simulink model "TSR_Scenario_002_cs"  (R2014b)
settings: Solver=ode5  SolverMode=SingleTasking  StartTime=0.0  StopTime=inf  FixedStep=1/100  RelTol=1e-3
PreLoadFcn:
  | mbxruntime.callbacks.PreLoadFcn(bdroot);
  | check_NUTS_defined;
  | 
  | assignin('base',['model_closed_' bdroot],false);
  | 
  | addpath('../includes_TSR/includes_TSR');
  | 
  | switch version('-release')
  | case {'2010a', '2010b', '2011a'}
  | addpath('../includes_TSR/ML2010b');
  | otherwise
  | addpath('../includes_TSR/ML2011b');
  | end
PostLoadFcn:
  | mbxruntime.callbacks.PostLoadFcn(bdroot);
InitFcn:
  | mbxruntime.callbacks.InitFcn(bdroot);;
  | 
  | addpath('..\includes_TSR');
StartFcn:
  | mbxruntime.callbacks.StartFcn(bdroot);
StopFcn:
  | mbxruntime.callbacks.StopFcn(bdroot);
model workspace: external: MAT-File .\TSR_Scenario_002_cs_hws.mat (data not in the file)
undefined symbols (not defined in the file or in its folder): InitImageOutputDir, mbxruntime, OrientationPitch, OrientationRoll, PositionX, PositionY, PositionZ, tabledata, warningInitialVelocity, x0
undefined symbols (not defined in the file): SteeringColumn, SteeringWheel, TSR_Scenario_002_cs_003e47b1b59594b6, TSR_Scenario_002_cs_023e87a31011dc74, TSR_Scenario_002_cs_048cb8409c90d9c6, TSR_Scenario_002_cs_106a0284aafa53e6, TSR_Scenario_002_cs_195b368d22a7f172, TSR_Scenario_002_cs_1e339fa5d680f213, TSR_Scenario_002_cs_26196a9fb104f950, TSR_Scenario_002_cs_261a709f6f453598, TSR_Scenario_002_cs_2ac3337370d0049d, TSR_Scenario_002_cs_2dc51e6a68b01b00, TSR_Scenario_002_cs_3460ff54d38ab2e2, TSR_Scenario_002_cs_42ea7d6e56bd6005, TSR_Scenario_002_cs_4dd419d6d2b56fc2, TSR_Scenario_002_cs_5316a21de09dff2f, TSR_Scenario_002_cs_538caacf3455966d, TSR_Scenario_002_cs_5b2cfdbcfc80811f, TSR_Scenario_002_cs_5ce0eafbb7a2dce7, TSR_Scenario_002_cs_62cdbf45c6f8824a, TSR_Scenario_002_cs_6bebc368eedff0bc, TSR_Scenario_002_cs_6d26481da4ed7e29, TSR_Scenario_002_cs_70c7e369ce6550e0, TSR_Scenario_002_cs_7a63051a1f311451, TSR_Scenario_002_cs_7d7dc8405f613c6d, TSR_Scenario_002_cs_7f65e296173485e8, TSR_Scenario_002_cs_87183cf6ff7bb4b6, TSR_Scenario_002_cs_8921b0da7ab80865, TSR_Scenario_002_cs_9495ce3a76763d1f, TSR_Scenario_002_cs_a679806a2fdc8099, TSR_Scenario_002_cs_Actros_1860_1_Path_pathUniqueID, TSR_Scenario_002_cs_Actros_2541_1_Path_pathUniqueID, TSR_Scenario_002_cs_Actros_2541_3_Path_pathUniqueID, TSR_Scenario_002_cs_Actros_2541_4_Path_pathUniqueID, TSR_Scenario_002_cs_adf24c93a9de8a4e, TSR_Scenario_002_cs_Audi_A8_1_Dynamics_Simple_initialPitch, TSR_Scenario_002_cs_Audi_A8_1_Dynamics_Simple_initialRoll, TSR_Scenario_002_cs_Audi_A8_1_Dynamics_Simple_initialX, TSR_Scenario_002_cs_Audi_A8_1_Dynamics_Simple_initialY, TSR_Scenario_002_cs_Audi_A8_1_Dynamics_Simple_initialYaw, TSR_Scenario_002_cs_Audi_A8_1_Dynamics_Simple_initialZ, TSR_Scenario_002_cs_b136c6ccb55f77db, TSR_Scenario_002_cs_ba4f809714c282b7, TSR_Scenario_002_cs_BMW_X5_1_Path_pathUniqueID, TSR_Scenario_002_cs_BMW_X5_1_SpeedProfile_speedProfileUniqueID, TSR_Scenario_002_cs_BMW_X5_2_Path_pathUniqueID, TSR_Scenario_002_cs_BMW_X5_2_SpeedProfile_speedProfileUniqueID, TSR_Scenario_002_cs_Citroen_C3_1_Path_pathUniqueID, TSR_Scenario_002_cs_Citroen_C3_2_Path_pathUniqueID, TSR_Scenario_002_cs_d8f275339b7082cf, TSR_Scenario_002_cs_Daf_95_1_Path_pathUniqueID, TSR_Scenario_002_cs_Daf_95_1_SpeedProfile_speedProfileUniqueID, TSR_Scenario_002_cs_dc019741510ce2f2, TSR_Scenario_002_cs_fdbc8aabe460b27c, TSR_Scenario_002_cs_Fiat_Bravo_1_Path_pathUniqueID, TSR_Scenario_002_cs_Ford_Fiesta_1_Path_pathUniqueID, TSR_Scenario_002_cs_Honda_Pan_European_1_Path_pathUniqueID, TSR_Scenario_002_cs_Mazda_RX8_1_Path_pathUniqueID, TSR_Scenario_002_cs_Nissan_Cabstar_1_Path_pathUniqueID, TSR_Scenario_002_cs_Nissan_Cabstar_2_Path_pathUniqueID ... (+9)
libraries: simulink_extras x82, simulink x23, PreScanSimulinkLibrary x11
(part 21 of 39)

== system TSR_Scenario_002_cs/HighwayOverhang_6/VISUMatrixSign_Mux ==
  MatrixSign_19 : Inport
  MatrixSign_20 : Inport  Port=2
  MatrixSign_19_Conversion : DataTypeConversion
  MatrixSign_19_InitialResource : Constant
  MatrixSign_19_Switch : Switch  Criteria=u2 ~= 0
  MatrixSign_20_Conversion : DataTypeConversion
  MatrixSign_20_InitialResource : Constant
  MatrixSign_20_Switch : Switch  Criteria=u2 ~= 0
  SubMuxMatrixSign : Mux  Inputs=2
  MatrixSigns : Outport
  wires:
  SubMuxMatrixSign/1 -> MatrixSigns/1
  MatrixSign_19/1 -> MatrixSign_19_Switch/1, MatrixSign_19_Switch/2
  MatrixSign_19_InitialResource/1 -> MatrixSign_19_Switch/3
  MatrixSign_19_Switch/1 -> MatrixSign_19_Conversion/1
  MatrixSign_19_Conversion/1 -> SubMuxMatrixSign/1
  MatrixSign_20/1 -> MatrixSign_20_Switch/1, MatrixSign_20_Switch/2
  MatrixSign_20_InitialResource/1 -> MatrixSign_20_Switch/3
  MatrixSign_20_Switch/1 -> MatrixSign_20_Conversion/1
  MatrixSign_20_Conversion/1 -> SubMuxMatrixSign/2

== system TSR_Scenario_002_cs/HighwayOverhang_7/VISUMatrixSignLights_Mux ==
  MatrixSign_4 : Inport  Tag=inport/MatrixSign_4  PortDimensions=4  SampleTime=1/100  BusOutputAsStruct=on
  MatrixSign_45 : Inport  Tag=inport/MatrixSign_45  Port=2  PortDimensions=4  SampleTime=1/100  BusOutputAsStruct=on
  MuxVisuLights : Mux  Inputs=2
  VISUMatrixSignLights_HighwayOverhang_7 : Outport  Tag=outport/VisuMatrixSignLights  SampleTime=1/100
  wires:
  MuxVisuLights/1 -> VISUMatrixSignLights_HighwayOverhang_7/1
  MatrixSign_4/1 -> MuxVisuLights/1
  MatrixSign_45/1 -> MuxVisuLights/2

== system TSR_Scenario_002_cs/HighwayOverhang_7/VISUMatrixSign_Mux ==
  MatrixSign_4 : Inport
  MatrixSign_45 : Inport  Port=2
  MatrixSign_45_Conversion : DataTypeConversion
  MatrixSign_45_InitialResource : Constant  Value=15
  MatrixSign_45_Switch : Switch  Criteria=u2 ~= 0
  MatrixSign_4_Conversion : DataTypeConversion
  MatrixSign_4_InitialResource : Constant  Value=15
  MatrixSign_4_Switch : Switch  Criteria=u2 ~= 0
  SubMuxMatrixSign : Mux  Inputs=2
  MatrixSigns : Outport
  wires:
  SubMuxMatrixSign/1 -> MatrixSigns/1
  MatrixSign_4/1 -> MatrixSign_4_Switch/1, MatrixSign_4_Switch/2
  MatrixSign_4_InitialResource/1 -> MatrixSign_4_Switch/3
  MatrixSign_4_Switch/1 -> MatrixSign_4_Conversion/1
  MatrixSign_4_Conversion/1 -> SubMuxMatrixSign/1
  MatrixSign_45/1 -> MatrixSign_45_Switch/1, MatrixSign_45_Switch/2
  MatrixSign_45_InitialResource/1 -> MatrixSign_45_Switch/3
  MatrixSign_45_Switch/1 -> MatrixSign_45_Conversion/1
  MatrixSign_45_Conversion/1 -> SubMuxMatrixSign/2

== system TSR_Scenario_002_cs/HighwayOverhang_8/VISUMatrixSignLights_Mux ==
  MatrixSign_15 : Inport  Tag=inport/MatrixSign_15  PortDimensions=4  SampleTime=1/100  BusOutputAsStruct=on
  MatrixSign_16 : Inport  Tag=inport/MatrixSign_16  Port=2  PortDimensions=4  SampleTime=1/100  BusOutputAsStruct=on
  MuxVisuLights : Mux  Inputs=2
  VISUMatrixSignLights_HighwayOverhang_8 : Outport  Tag=outport/VisuMatrixSignLights  SampleTime=1/100
  wires:
  MuxVisuLights/1 -> VISUMatrixSignLights_HighwayOverhang_8/1
  MatrixSign_15/1 -> MuxVisuLights/1
  MatrixSign_16/1 -> MuxVisuLights/2

== system TSR_Scenario_002_cs/HighwayOverhang_8/VISUMatrixSign_Mux ==
  MatrixSign_15 : Inport
  MatrixSign_16 : Inport  Port=2
  MatrixSign_15_Conversion : DataTypeConversion
  MatrixSign_15_InitialResource : Constant
  MatrixSign_15_Switch : Switch  Criteria=u2 ~= 0
  MatrixSign_16_Conversion : DataTypeConversion
  MatrixSign_16_InitialResource : Constant
  MatrixSign_16_Switch : Switch  Criteria=u2 ~= 0
  SubMuxMatrixSign : Mux  Inputs=2
  MatrixSigns : Outport
  wires:
  SubMuxMatrixSign/1 -> MatrixSigns/1
  MatrixSign_15/1 -> MatrixSign_15_Switch/1, MatrixSign_15_Switch/2
  MatrixSign_15_InitialResource/1 -> MatrixSign_15_Switch/3
  MatrixSign_15_Switch/1 -> MatrixSign_15_Conversion/1
  MatrixSign_15_Conversion/1 -> SubMuxMatrixSign/1
  MatrixSign_16/1 -> MatrixSign_16_Switch/1, MatrixSign_16_Switch/2
  MatrixSign_16_InitialResource/1 -> MatrixSign_16_Switch/3
  MatrixSign_16_Switch/1 -> MatrixSign_16_Conversion/1
  MatrixSign_16_Conversion/1 -> SubMuxMatrixSign/2

== system TSR_Scenario_002_cs/HighwayOverhang_9/VISUMatrixSignLights_Mux ==
  MatrixSign_47 : Inport  Tag=inport/MatrixSign_47  PortDimensions=4  SampleTime=1/100  BusOutputAsStruct=on
  MatrixSign_6 : Inport  Tag=inport/MatrixSign_6  Port=2  PortDimensions=4  SampleTime=1/100  BusOutputAsStruct=on
  MuxVisuLights : Mux  Inputs=2
  VISUMatrixSignLights_HighwayOverhang_9 : Outport  Tag=outport/VisuMatrixSignLights  SampleTime=1/100
  wires:
  MuxVisuLights/1 -> VISUMatrixSignLights_HighwayOverhang_9/1
  MatrixSign_47/1 -> MuxVisuLights/1
  MatrixSign_6/1 -> MuxVisuLights/2

== system TSR_Scenario_002_cs/HighwayOverhang_9/VISUMatrixSign_Mux ==
  MatrixSign_6 : Inport
  MatrixSign_47 : Inport  Port=2
  MatrixSign_47_Conversion : DataTypeConversion
  MatrixSign_47_InitialResource : Constant  Value=13
  MatrixSign_47_Switch : Switch  Criteria=u2 ~= 0
  MatrixSign_6_Conversion : DataTypeConversion
  MatrixSign_6_InitialResource : Constant  Value=13
  MatrixSign_6_Switch : Switch  Criteria=u2 ~= 0
  SubMuxMatrixSign : Mux  Inputs=2
  MatrixSigns : Outport
  wires:
  SubMuxMatrixSign/1 -> MatrixSigns/1
  MatrixSign_6/1 -> MatrixSign_6_Switch/1, MatrixSign_6_Switch/2
  MatrixSign_6_InitialResource/1 -> MatrixSign_6_Switch/3
  MatrixSign_6_Switch/1 -> MatrixSign_6_Conversion/1
  MatrixSign_6_Conversion/1 -> SubMuxMatrixSign/1
  MatrixSign_47/1 -> MatrixSign_47_Switch/1, MatrixSign_47_Switch/2
  MatrixSign_47_InitialResource/1 -> MatrixSign_47_Switch/3
  MatrixSign_47_Switch/1 -> MatrixSign_47_Conversion/1
  MatrixSign_47_Conversion/1 -> SubMuxMatrixSign/2

== system TSR_Scenario_002_cs/Honda_Pan_European_1/SELF_Demux ==
  SELF : Inport  OutDataTypeStr=Bus: PRESCAN_SELFSENSORDATA
  Bus Selector : BusSelector  OutputSignals=PositionX,PositionY,PositionZ,OrientationRoll,OrientationPitch,OrientationYaw,Velocity,Yaw_rate,Lat,Long,Alt
  Demux2 : Demux  Outputs=3
  Gain : Gain  Gain=180/pi
  Gain1 : Gain  Gain=180/pi
  Vector Concatenate1 : Concatenate  NumInputs=3
  compas converter : Subsystem
  x [m] : Outport
  y [m] : Outport  Port=2
  z [m] : Outport  Port=3
  rotx [deg] : Outport  Port=4
  roty [deg] : Outport  Port=5
  rotz [deg] : Outport  Port=6
  GPS lat [deg] : Outport  Port=7
  GPS long [deg] : Outport  Port=8
  GPS alt [m] : Outport  Port=9
  velocity [m/s] : Outport  Port=10
  heading [deg] : Outport  Port=11
  yaw rate [deg/s] : Outport  Port=12
  wires:
  Bus Selector/11 -> GPS alt [m]/1  "<Alt>"
  Bus Selector/10 -> GPS long [deg]/1  "<Long>"
  Bus Selector/9 -> GPS lat [deg]/1  "<Lat>"
  Bus Selector/8 -> Gain1/1  "<Yaw_rate>"
  Bus Selector/7 -> velocity [m/s]/1  "<Velocity>"
  Bus Selector/6 -> compas converter/1(rotz [rad]), Vector Concatenate1/3  "<OrientationYaw>"
  Bus Selector/5 -> Vector Concatenate1/2  "<OrientationPitch>"
  Bus Selector/4 -> Vector Concatenate1/1  "<OrientationRoll>"
  Vector Concatenate1/1 -> Gain/1
  Bus Selector/3 -> z [m]/1  "<PositionZ>"
  Bus Selector/2 -> y [m]/1  "<PositionY>"
  Bus Selector/1 -> x [m]/1  "<PositionX>"
  SELF/1 -> Bus Selector/1
  Gain/1 -> Demux2/1
  Demux2/1 -> rotx [deg]/1
  Demux2/2 -> roty [deg]/1
  Demux2/3 -> rotz [deg]/1
  compas converter/1(heading [deg]) -> heading [deg]/1
  Gain1/1 -> yaw rate [deg/s]/1

== system TSR_Scenario_002_cs/Male_RegularAni_1/Animation ==
  In1 : Inport
  Bus Creator : BusCreator  Inputs=2  OutDataTypeStr=Bus: PRESCAN_ANIMACTUATORDATA  NonVirtualBus=on
  Bus Selector : BusSelector  OutputSignals=VelocityX,VelocityY,VelocityZ
  Data Type Conversion : DataTypeConversion  OutDataTypeStr=int32
  Mux : Mux  Inputs=3
  Product : Product  RndMeth=Zero
  RunningScale : Constant  Value=RunningScale
  Switch : Switch  Threshold=2
  WalkingScale : Constant  Value=WalkingScale
  animation mode : Subsystem
  elapsed track : Subsystem
  Out1 : Outport
  wires:
  Switch/1 -> Product/1
  WalkingScale/1 -> Switch/3
  RunningScale/1 -> Switch/1
  elapsed track/1(s) -> Product/2  "Time"
  Product/1 -> Bus Creator/2  "Time"
  Mux/1 -> elapsed track/1(vel), animation mode/1(vel)
  Bus Selector/1 -> Mux/1  "<VelocityX>"
  Bus Selector/2 -> Mux/2  "<VelocityY>"
  Bus Selector/3 -> Mux/3  "<VelocityZ>"
  animation mode/1(mode) -> Switch/2, Data Type Conversion/1
  In1/1 -> Bus Selector/1
  Bus Creator/1 -> Out1/1
  Data Type Conversion/1 -> Bus Creator/1  "Index"

== system TSR_Scenario_002_cs/Male_RegularAni_1/Dynamics_Empty ==
  note: For state mode 'Dynamic' positions
      | are not taken into account, as they
      | are computed by integrating velocity.
      | Click annotation for Help.
  Ground_{1..9} (9 alike) : Ground
  MuxState : Subsystem  Tag=mux/State  mask(Empty Dynamics State Block){positioningmode=on, TimeStep=1/100}
      mask prompts: positioningmode "Positioning Mode"; TimeStep "Auto Assigned: Time Step [s]"
      mask help:
      | Build the state of an actor based on user input.
      | The user can either use positioning mode or dynamics mode.
      | - When using positioning mode the position and orientation of the actor are set directly based on the input. Expected input is relative to the initial position and orientation of the actor. It's also possible to specify the velocity of the actor, though this input isn't used, only passed on.
      | - When using dynamics mode the position input is ignored. Expected input is velocity and orientation. The velocity is relative the current orientation of the actor, while orientation is relative to its initial orientation. The position of the actor is calculated based on the velocity and orientation given.
      settings: DeleteFcn=PreScanBlockDeleteFcn;
  STATE_Male_RegularAni_1 : Subsystem  Tag=mux/StatePort  Priority=0  LoadFcn=load PrescanStateActuatorData  mask(PreScan Sink Block: State){x0=TSR_Scenario_002_cs_003e47b1b59594b6, y0=TSR_Scenario_002_cs_6d26481da4ed7e29, z0=TSR_Scenario_002_cs_7f65e296173485e8, Roll0=TSR_Scenario_002_cs_8921b0da7ab80865, Pitch0=TSR_Scenario_002_cs_a679806a2fdc8099, Yaw0=TSR_Scenario_002_cs_dc019741510ce2f2, TimeStep=1/100}
      mask prompts: x0 "Ini x-position VEHICLE wrt GLOBAL axis system [m]"; y0 "Ini y-position VEHICLE wrt GLOBAL axis system [m]"; z0 "Ini z-position VEHICLE wrt GLOBAL axis system [m]"; Roll0 "Ini roll-angle BODY wrt VEHICLE axis system [deg]"; Pitch0 "Ini pitch-angle BODY wrt VEHICLE axis system [deg]"; Yaw0 "Ini yaw-angle VEHICLE wrt GLOBAL axis system [deg]"; TimeStep "Auto-Assigned: Upload Period [s]"
      mask help:
      | The Actor State contains a vector signal of size (9x1), containing the following signals:
      |
      | -  Position                  (x,y,z)                                     [m]
      | -  Velocity                  (vx,vy,vz)                               [m/s]
      | -  Angles                    (Roll, Pitch, Yaw)                   [rad]
      |
      | The Actor state is defined in the global axis system.
      | The state is superponed on the Initial position defined in the GUI.
      |
      | For more information, please click Help.
      settings: DeleteFcn=PreScanBlockDeleteFcn;
      mask Help: eval('openHelp(222)')
      mask Display: image(imread('State.png'))
  State : Outport  Tag=outport/StateOutport  SampleTime=1/100
  wires:
  MuxState/1(state) -> STATE_Male_RegularAni_1/1(State)
  STATE_Male_RegularAni_1/1(StateBus) -> State/1
  Ground_1/1 -> MuxState/1(x [m])
  Ground_2/1 -> MuxState/2(y [m])
  Ground_3/1 -> MuxState/3(z [m])
  Ground_4/1 -> MuxState/4(dx [m/s])
  Ground_5/1 -> MuxState/5(dy [m/s])
  Ground_6/1 -> MuxState/6(dz [m/s])
  Ground_7/1 -> MuxState/7(R [rad])
  Ground_8/1 -> MuxState/8(P [rad])
  Ground_9/1 -> MuxState/9(Y [rad])

== system TSR_Scenario_002_cs/Male_RegularAni_1/SELF_Demux ==
  SELF : Inport  OutDataTypeStr=Bus: PRESCAN_SELFSENSORDATA
  Bus Selector : BusSelector  OutputSignals=PositionX,PositionY,PositionZ,OrientationRoll,OrientationPitch,OrientationYaw,Velocity,Yaw_rate,Lat,Long,Alt
  Demux2 : Demux  Outputs=3
  Gain : Gain  Gain=180/pi
  Gain1 : Gain  Gain=180/pi
  Vector Concatenate1 : Concatenate  NumInputs=3
  compas converter : Subsystem
  x [m] : Outport
  y [m] : Outport  Port=2
  z [m] : Outport  Port=3
  rotx [deg] : Outport  Port=4
  roty [deg] : Outport  Port=5
  rotz [deg] : Outport  Port=6
  GPS lat [deg] : Outport  Port=7
  GPS long [deg] : Outport  Port=8
  GPS alt [m] : Outport  Port=9
  velocity [m/s] : Outport  Port=10
  heading [deg] : Outport  Port=11
  yaw rate [deg/s] : Outport  Port=12
  wires:
  Bus Selector/11 -> GPS alt [m]/1  "<Alt>"
  Bus Selector/10 -> GPS long [deg]/1  "<Long>"
  Bus Selector/9 -> GPS lat [deg]/1  "<Lat>"
  Bus Selector/8 -> Gain1/1  "<Yaw_rate>"
  Bus Selector/7 -> velocity [m/s]/1  "<Velocity>"
  Bus Selector/6 -> compas converter/1(rotz [rad]), Vector Concatenate1/3  "<OrientationYaw>"
  Bus Selector/5 -> Vector Concatenate1/2  "<OrientationPitch>"
  Bus Selector/4 -> Vector Concatenate1/1  "<OrientationRoll>"
  Vector Concatenate1/1 -> Gain/1
  Bus Selector/3 -> z [m]/1  "<PositionZ>"
  Bus Selector/2 -> y [m]/1  "<PositionY>"
  Bus Selector/1 -> x [m]/1  "<PositionX>"
  SELF/1 -> Bus Selector/1
  Gain/1 -> Demux2/1
  Demux2/1 -> rotx [deg]/1
  Demux2/2 -> roty [deg]/1
  Demux2/3 -> rotz [deg]/1
  compas converter/1(heading [deg]) -> heading [deg]/1
  Gain1/1 -> yaw rate [deg/s]/1

== system TSR_Scenario_002_cs/Male_RegularAni_1/VISUColorRegion_Lower_Body_Mux ==
  RGB [-,-,-] : Inport
  Bus Creator : BusCreator  OutDataTypeStr=Bus: PRESCAN_COLOR_DATA  NonVirtualBus=on
  Constant : Constant  Value=255  OutDataTypeStr=uint8
  Data Type Conversion : DataTypeConversion  OutDataTypeStr=uint8
  Data Type Conversion1 : DataTypeConversion  OutDataTypeStr=uint8
  Data Type Conversion2 : DataTypeConversion  OutDataTypeStr=uint8
  Demux : Demux  Outputs=3
  ColorRegion : Outport  OutDataTypeStr=Bus: PRESCAN_COLOR_DATA  PortDimensions=1
  wires:
  Constant/1 -> Bus Creator/4  "A"
  Data Type Conversion2/1 -> Bus Creator/3  "B"
  Data Type Conversion1/1 -> Bus Creator/2  "G"
  Data Type Conversion/1 -> Bus Creator/1  "R"
  Demux/3 -> Data Type Conversion2/1  "B"
  Demux/2 -> Data Type Conversion1/1  "G"
  Demux/1 -> Data Type Conversion/1  "R"
  RGB [-,-,-]/1 -> Demux/1
  Bus Creator/1 -> ColorRegion/1

== system TSR_Scenario_002_cs/Male_RegularAni_1/VISUColorRegion_Shoes_Mux ==
  RGB [-,-,-] : Inport
  Bus Creator : BusCreator  OutDataTypeStr=Bus: PRESCAN_COLOR_DATA  NonVirtualBus=on
  Constant : Constant  Value=255  OutDataTypeStr=uint8
  Data Type Conversion : DataTypeConversion  OutDataTypeStr=uint8
  Data Type Conversion1 : DataTypeConversion  OutDataTypeStr=uint8
  Data Type Conversion2 : DataTypeConversion  OutDataTypeStr=uint8
  Demux : Demux  Outputs=3
  ColorRegion : Outport  OutDataTypeStr=Bus: PRESCAN_COLOR_DATA  PortDimensions=1
  wires:
  Constant/1 -> Bus Creator/4  "A"
  Data Type Conversion2/1 -> Bus Creator/3  "B"
  Data Type Conversion1/1 -> Bus Creator/2  "G"
  Data Type Conversion/1 -> Bus Creator/1  "R"
  Demux/3 -> Data Type Conversion2/1  "B"
  Demux/2 -> Data Type Conversion1/1  "G"
  Demux/1 -> Data Type Conversion/1  "R"
  RGB [-,-,-]/1 -> Demux/1
  Bus Creator/1 -> ColorRegion/1

== system TSR_Scenario_002_cs/Male_RegularAni_1/VISUColorRegion_Upper_Body_Mux ==
  RGB [-,-,-] : Inport
  Bus Creator : BusCreator  OutDataTypeStr=Bus: PRESCAN_COLOR_DATA  NonVirtualBus=on
  Constant : Constant  Value=255  OutDataTypeStr=uint8
  Data Type Conversion : DataTypeConversion  OutDataTypeStr=uint8
  Data Type Conversion1 : DataTypeConversion  OutDataTypeStr=uint8
  Data Type Conversion2 : DataTypeConversion  OutDataTypeStr=uint8
  Demux : Demux  Outputs=3
  ColorRegion : Outport  OutDataTypeStr=Bus: PRESCAN_COLOR_DATA  PortDimensions=1
  wires:
  Constant/1 -> Bus Creator/4  "A"
  Data Type Conversion2/1 -> Bus Creator/3  "B"
  Data Type Conversion1/1 -> Bus Creator/2  "G"
  Data Type Conversion/1 -> Bus Creator/1  "R"
  Demux/3 -> Data Type Conversion2/1  "B"
  Demux/2 -> Data Type Conversion1/1  "G"
  Demux/1 -> Data Type Conversion/1  "R"
  RGB [-,-,-]/1 -> Demux/1
  Bus Creator/1 -> ColorRegion/1

== system TSR_Scenario_002_cs/Mazda_RX8_1/SELF_Demux ==
  SELF : Inport  OutDataTypeStr=Bus: PRESCAN_SELFSENSORDATA
  Bus Selector : BusSelector  OutputSignals=PositionX,PositionY,PositionZ,OrientationRoll,OrientationPitch,OrientationYaw,Velocity,Yaw_rate,Lat,Long,Alt
  Demux2 : Demux  Outputs=3
  Gain : Gain  Gain=180/pi
  Gain1 : Gain  Gain=180/pi
  Vector Concatenate1 : Concatenate  NumInputs=3
  compas converter : Subsystem
  x [m] : Outport
  y [m] : Outport  Port=2
  z [m] : Outport  Port=3
  rotx [deg] : Outport  Port=4
  roty [deg] : Outport  Port=5
  rotz [deg] : Outport  Port=6
  GPS lat [deg] : Outport  Port=7
  GPS long [deg] : Outport  Port=8
  GPS alt [m] : Outport  Port=9
  velocity [m/s] : Outport  Port=10
  heading [deg] : Outport  Port=11
  yaw rate [deg/s] : Outport  Port=12
  wires:
  Bus Selector/11 -> GPS alt [m]/1  "<Alt>"
  Bus Selector/10 -> GPS long [deg]/1  "<Long>"
  Bus Selector/9 -> GPS lat [deg]/1  "<Lat>"
  Bus Selector/8 -> Gain1/1  "<Yaw_rate>"
  Bus Selector/7 -> velocity [m/s]/1  "<Velocity>"
  Bus Selector/6 -> compas converter/1(rotz [rad]), Vector Concatenate1/3  "<OrientationYaw>"
  Bus Selector/5 -> Vector Concatenate1/2  "<OrientationPitch>"
  Bus Selector/4 -> Vector Concatenate1/1  "<OrientationRoll>"
  Vector Concatenate1/1 -> Gain/1
  Bus Selector/3 -> z [m]/1  "<PositionZ>"
  Bus Selector/2 -> y [m]/1  "<PositionY>"
  Bus Selector/1 -> x [m]/1  "<PositionX>"
  SELF/1 -> Bus Selector/1
  Gain/1 -> Demux2/1
  Demux2/1 -> rotx [deg]/1
  Demux2/2 -> roty [deg]/1
  Demux2/3 -> rotz [deg]/1
  compas converter/1(heading [deg]) -> heading [deg]/1
  Gain1/1 -> yaw rate [deg/s]/1

== system TSR_Scenario_002_cs/Nissan_Cabstar_1/Brake_light_left_Mux ==
  MSCD [Cd] : Inport
  Position (xyz) [m] : Inport  Port=2
  Orientation (RPY) [deg] : Inport  Port=3
  Color [-] : Inport  Port=4
  TextureResourceID [-] : Inport  Port=5
  Bus Creator : BusCreator  Inputs='Intensity','Position','Orientation','Color','TextureResourceID'  OutDataTypeStr=Bus: PRESCAN_VISULIGHTACTUATOR_DATA  NonVirtualBus=on
  Bus Creator1 : BusCreator  Inputs=3  OutDataTypeStr=Bus: PRESCAN_RGB_DATA  NonVirtualBus=on
  Bus Creator2 : BusCreator  Inputs=3  OutDataTypeStr=Bus: PRESCAN_RPY_DATA  NonVirtualBus=on
  Bus Creator3 : BusCreator  Inputs=3  OutDataTypeStr=Bus: PRESCAN_XYZ_DATA  NonVirtualBus=on
  Data Type Conversion : DataTypeConversion  OutDataTypeStr=int32  RndMeth=Nearest
  Degrees to Radians : simulink_extras/Transformations/Degrees to Radians
  Demux : Demux  Outputs=3
  Demux1 : Demux  Outputs=3
  Demux2 : Demux  Outputs=3
  Lights : Outport
  wires:
  TextureResourceID [-]/1 -> Data Type Conversion/1  "TextureResourceID"
  MSCD [Cd]/1 -> Bus Creator/1  "Intensity"
  Bus Creator/1 -> Lights/1
  Demux/1 -> Bus Creator1/1  "R"
  Demux/2 -> Bus Creator1/2  "G"
  Demux/3 -> Bus Creator1/3  "B"
  Color [-]/1 -> Demux/1  "Color"
  Bus Creator1/1 -> Bus Creator/4  "Color"
  Demux1/1 -> Bus Creator2/1  "Roll"
  Demux1/2 -> Bus Creator2/2  "Pitch"
  Demux1/3 -> Bus Creator2/3  "Yaw"
  Orientation (RPY) [deg]/1 -> Degrees to Radians/1  "Orientation"
  Bus Creator2/1 -> Bus Creator/3  "Orientation"
  Demux2/1 -> Bus Creator3/1  "X"
  Demux2/2 -> Bus Creator3/2  "Y"
  Demux2/3 -> Bus Creator3/3  "Z"
  Position (xyz) [m]/1 -> Demux2/1  "Position"
  Bus Creator3/1 -> Bus Creator/2  "Position"
  Data Type Conversion/1 -> Bus Creator/5  "TextureResourceID"
  Degrees to Radians/1 -> Demux1/1

== system TSR_Scenario_002_cs/Nissan_Cabstar_1/Brake_light_right_Mux ==
  MSCD [Cd] : Inport
  Position (xyz) [m] : Inport  Port=2
  Orientation (RPY) [deg] : Inport  Port=3
  Color [-] : Inport  Port=4
  TextureResourceID [-] : Inport  Port=5
  Bus Creator : BusCreator  Inputs='Intensity','Position','Orientation','Color','TextureResourceID'  OutDataTypeStr=Bus: PRESCAN_VISULIGHTACTUATOR_DATA  NonVirtualBus=on
  Bus Creator1 : BusCreator  Inputs=3  OutDataTypeStr=Bus: PRESCAN_RGB_DATA  NonVirtualBus=on
  Bus Creator2 : BusCreator  Inputs=3  OutDataTypeStr=Bus: PRESCAN_RPY_DATA  NonVirtualBus=on
  Bus Creator3 : BusCreator  Inputs=3  OutDataTypeStr=Bus: PRESCAN_XYZ_DATA  NonVirtualBus=on
  Data Type Conversion : DataTypeConversion  OutDataTypeStr=int32  RndMeth=Nearest
  Degrees to Radians : simulink_extras/Transformations/Degrees to Radians
  Demux : Demux  Outputs=3
  Demux1 : Demux  Outputs=3
  Demux2 : Demux  Outputs=3
  Lights : Outport
  wires:
  TextureResourceID [-]/1 -> Data Type Conversion/1  "TextureResourceID"
  MSCD [Cd]/1 -> Bus Creator/1  "Intensity"
  Bus Creator/1 -> Lights/1
  Demux/1 -> Bus Creator1/1  "R"
  Demux/2 -> Bus Creator1/2  "G"
  Demux/3 -> Bus Creator1/3  "B"
  Color [-]/1 -> Demux/1  "Color"
  Bus Creator1/1 -> Bus Creator/4  "Color"
  Demux1/1 -> Bus Creator2/1  "Roll"
  Demux1/2 -> Bus Creator2/2  "Pitch"
  Demux1/3 -> Bus Creator2/3  "Yaw"
  Orientation (RPY) [deg]/1 -> Degrees to Radians/1  "Orientation"
  Bus Creator2/1 -> Bus Creator/3  "Orientation"
  Demux2/1 -> Bus Creator3/1  "X"
  Demux2/2 -> Bus Creator3/2  "Y"
  Demux2/3 -> Bus Creator3/3  "Z"
  Position (xyz) [m]/1 -> Demux2/1  "Position"
  Bus Creator3/1 -> Bus Creator/2  "Position"
  Data Type Conversion/1 -> Bus Creator/5  "TextureResourceID"
  Degrees to Radians/1 -> Demux1/1

== system TSR_Scenario_002_cs/Nissan_Cabstar_1/Indicator_front_left_Mux ==
  MSCD [Cd] : Inport
  Position (xyz) [m] : Inport  Port=2
  Orientation (RPY) [deg] : Inport  Port=3
  Color [-] : Inport  Port=4
  TextureResourceID [-] : Inport  Port=5
  Bus Creator : BusCreator  Inputs='Intensity','Position','Orientation','Color','TextureResourceID'  OutDataTypeStr=Bus: PRESCAN_VISULIGHTACTUATOR_DATA  NonVirtualBus=on
  Bus Creator1 : BusCreator  Inputs=3  OutDataTypeStr=Bus: PRESCAN_RGB_DATA  NonVirtualBus=on
  Bus Creator2 : BusCreator  Inputs=3  OutDataTypeStr=Bus: PRESCAN_RPY_DATA  NonVirtualBus=on
  Bus Creator3 : BusCreator  Inputs=3  OutDataTypeStr=Bus: PRESCAN_XYZ_DATA  NonVirtualBus=on
  Data Type Conversion : DataTypeConversion  OutDataTypeStr=int32  RndMeth=Nearest
  Degrees to Radians : simulink_extras/Transformations/Degrees to Radians
  Demux : Demux  Outputs=3
  Demux1 : Demux  Outputs=3
  Demux2 : Demux  Outputs=3
  Lights : Outport
  wires:
  TextureResourceID [-]/1 -> Data Type Conversion/1  "TextureResourceID"
  MSCD [Cd]/1 -> Bus Creator/1  "Intensity"
  Bus Creator/1 -> Lights/1
  Demux/1 -> Bus Creator1/1  "R"
  Demux/2 -> Bus Creator1/2  "G"
  Demux/3 -> Bus Creator1/3  "B"
  Color [-]/1 -> Demux/1  "Color"
  Bus Creator1/1 -> Bus Creator/4  "Color"
  Demux1/1 -> Bus Creator2/1  "Roll"
  Demux1/2 -> Bus Creator2/2  "Pitch"
  Demux1/3 -> Bus Creator2/3  "Yaw"
  Orientation (RPY) [deg]/1 -> Degrees to Radians/1  "Orientation"
  Bus Creator2/1 -> Bus Creator/3  "Orientation"
  Demux2/1 -> Bus Creator3/1  "X"
  Demux2/2 -> Bus Creator3/2  "Y"
  Demux2/3 -> Bus Creator3/3  "Z"
  Position (xyz) [m]/1 -> Demux2/1  "Position"
  Bus Creator3/1 -> Bus Creator/2  "Position"
  Data Type Conversion/1 -> Bus Creator/5  "TextureResourceID"
  Degrees to Radians/1 -> Demux1/1

== system TSR_Scenario_002_cs/Nissan_Cabstar_1/Indicator_front_right_Mux ==
  MSCD [Cd] : Inport
  Position (xyz) [m] : Inport  Port=2
  Orientation (RPY) [deg] : Inport  Port=3
  Color [-] : Inport  Port=4
  TextureResourceID [-] : Inport  Port=5
  Bus Creator : BusCreator  Inputs='Intensity','Position','Orientation','Color','TextureResourceID'  OutDataTypeStr=Bus: PRESCAN_VISULIGHTACTUATOR_DATA  NonVirtualBus=on
  Bus Creator1 : BusCreator  Inputs=3  OutDataTypeStr=Bus: PRESCAN_RGB_DATA  NonVirtualBus=on
  Bus Creator2 : BusCreator  Inputs=3  OutDataTypeStr=Bus: PRESCAN_RPY_DATA  NonVirtualBus=on
  Bus Creator3 : BusCreator  Inputs=3  OutDataTypeStr=Bus: PRESCAN_XYZ_DATA  NonVirtualBus=on
  Data Type Conversion : DataTypeConversion  OutDataTypeStr=int32  RndMeth=Nearest
  Degrees to Radians : simulink_extras/Transformations/Degrees to Radians
  Demux : Demux  Outputs=3
  Demux1 : Demux  Outputs=3
  Demux2 : Demux  Outputs=3
  Lights : Outport
  wires:
  TextureResourceID [-]/1 -> Data Type Conversion/1  "TextureResourceID"
  MSCD [Cd]/1 -> Bus Creator/1  "Intensity"
  Bus Creator/1 -> Lights/1
  Demux/1 -> Bus Creator1/1  "R"
  Demux/2 -> Bus Creator1/2  "G"
  Demux/3 -> Bus Creator1/3  "B"
  Color [-]/1 -> Demux/1  "Color"
  Bus Creator1/1 -> Bus Creator/4  "Color"
  Demux1/1 -> Bus Creator2/1  "Roll"
  Demux1/2 -> Bus Creator2/2  "Pitch"
  Demux1/3 -> Bus Creator2/3  "Yaw"
  Orientation (RPY) [deg]/1 -> Degrees to Radians/1  "Orientation"
  Bus Creator2/1 -> Bus Creator/3  "Orientation"
  Demux2/1 -> Bus Creator3/1  "X"
  Demux2/2 -> Bus Creator3/2  "Y"
  Demux2/3 -> Bus Creator3/3  "Z"
  Position (xyz) [m]/1 -> Demux2/1  "Position"
  Bus Creator3/1 -> Bus Creator/2  "Position"
  Data Type Conversion/1 -> Bus Creator/5  "TextureResourceID"
  Degrees to Radians/1 -> Demux1/1

== system TSR_Scenario_002_cs/Nissan_Cabstar_1/Indicator_rear_left_Mux ==
  MSCD [Cd] : Inport
  Position (xyz) [m] : Inport  Port=2
  Orientation (RPY) [deg] : Inport  Port=3
  Color [-] : Inport  Port=4
  TextureResourceID [-] : Inport  Port=5
  Bus Creator : BusCreator  Inputs='Intensity','Position','Orientation','Color','TextureResourceID'  OutDataTypeStr=Bus: PRESCAN_VISULIGHTACTUATOR_DATA  NonVirtualBus=on
  Bus Creator1 : BusCreator  Inputs=3  OutDataTypeStr=Bus: PRESCAN_RGB_DATA  NonVirtualBus=on
  Bus Creator2 : BusCreator  Inputs=3  OutDataTypeStr=Bus: PRESCAN_RPY_DATA  NonVirtualBus=on
  Bus Creator3 : BusCreator  Inputs=3  OutDataTypeStr=Bus: PRESCAN_XYZ_DATA  NonVirtualBus=on
  Data Type Conversion : DataTypeConversion  OutDataTypeStr=int32  RndMeth=Nearest
  Degrees to Radians : simulink_extras/Transformations/Degrees to Radians
  Demux : Demux  Outputs=3
  Demux1 : Demux  Outputs=3
  Demux2 : Demux  Outputs=3
  Lights : Outport
  wires:
  TextureResourceID [-]/1 -> Data Type Conversion/1  "TextureResourceID"
  MSCD [Cd]/1 -> Bus Creator/1  "Intensity"
  Bus Creator/1 -> Lights/1
  Demux/1 -> Bus Creator1/1  "R"
  Demux/2 -> Bus Creator1/2  "G"
  Demux/3 -> Bus Creator1/3  "B"
  Color [-]/1 -> Demux/1  "Color"
  Bus Creator1/1 -> Bus Creator/4  "Color"
  Demux1/1 -> Bus Creator2/1  "Roll"
  Demux1/2 -> Bus Creator2/2  "Pitch"
  Demux1/3 -> Bus Creator2/3  "Yaw"
  Orientation (RPY) [deg]/1 -> Degrees to Radians/1  "Orientation"
  Bus Creator2/1 -> Bus Creator/3  "Orientation"
  Demux2/1 -> Bus Creator3/1  "X"
  Demux2/2 -> Bus Creator3/2  "Y"
  Demux2/3 -> Bus Creator3/3  "Z"
  Position (xyz) [m]/1 -> Demux2/1  "Position"
  Bus Creator3/1 -> Bus Creator/2  "Position"
  Data Type Conversion/1 -> Bus Creator/5  "TextureResourceID"
  Degrees to Radians/1 -> Demux1/1

== system TSR_Scenario_002_cs/Nissan_Cabstar_1/Indicator_rear_right_Mux ==
  MSCD [Cd] : Inport
  Position (xyz) [m] : Inport  Port=2
  Orientation (RPY) [deg] : Inport  Port=3
  Color [-] : Inport  Port=4
  TextureResourceID [-] : Inport  Port=5
  Bus Creator : BusCreator  Inputs='Intensity','Position','Orientation','Color','TextureResourceID'  OutDataTypeStr=Bus: PRESCAN_VISULIGHTACTUATOR_DATA  NonVirtualBus=on
  Bus Creator1 : BusCreator  Inputs=3  OutDataTypeStr=Bus: PRESCAN_RGB_DATA  NonVirtualBus=on
  Bus Creator2 : BusCreator  Inputs=3  OutDataTypeStr=Bus: PRESCAN_RPY_DATA  NonVirtualBus=on
  Bus Creator3 : BusCreator  Inputs=3  OutDataTypeStr=Bus: PRESCAN_XYZ_DATA  NonVirtualBus=on
  Data Type Conversion : DataTypeConversion  OutDataTypeStr=int32  RndMeth=Nearest
  Degrees to Radians : simulink_extras/Transformations/Degrees to Radians
  Demux : Demux  Outputs=3
  Demux1 : Demux  Outputs=3
  Demux2 : Demux  Outputs=3
  Lights : Outport
  wires:
  TextureResourceID [-]/1 -> Data Type Conversion/1  "TextureResourceID"
  MSCD [Cd]/1 -> Bus Creator/1  "Intensity"
  Bus Creator/1 -> Lights/1
  Demux/1 -> Bus Creator1/1  "R"
  Demux/2 -> Bus Creator1/2  "G"
  Demux/3 -> Bus Creator1/3  "B"
  Color [-]/1 -> Demux/1  "Color"
  Bus Creator1/1 -> Bus Creator/4  "Color"
  Demux1/1 -> Bus Creator2/1  "Roll"
  Demux1/2 -> Bus Creator2/2  "Pitch"
  Demux1/3 -> Bus Creator2/3  "Yaw"
  Orientation (RPY) [deg]/1 -> Degrees to Radians/1  "Orientation"
  Bus Creator2/1 -> Bus Creator/3  "Orientation"
  Demux2/1 -> Bus Creator3/1  "X"
  Demux2/2 -> Bus Creator3/2  "Y"
  Demux2/3 -> Bus Creator3/3  "Z"
  Position (xyz) [m]/1 -> Demux2/1  "Position"
  Bus Creator3/1 -> Bus Creator/2  "Position"
  Data Type Conversion/1 -> Bus Creator/5  "TextureResourceID"
  Degrees to Radians/1 -> Demux1/1

== system TSR_Scenario_002_cs/Nissan_Cabstar_1/Indicator_side_left_Mux ==
  MSCD [Cd] : Inport
  Position (xyz) [m] : Inport  Port=2
  Orientation (RPY) [deg] : Inport  Port=3
  Color [-] : Inport  Port=4
  TextureResourceID [-] : Inport  Port=5
  Bus Creator : BusCreator  Inputs='Intensity','Position','Orientation','Color','TextureResourceID'  OutDataTypeStr=Bus: PRESCAN_VISULIGHTACTUATOR_DATA  NonVirtualBus=on
  Bus Creator1 : BusCreator  Inputs=3  OutDataTypeStr=Bus: PRESCAN_RGB_DATA  NonVirtualBus=on
  Bus Creator2 : BusCreator  Inputs=3  OutDataTypeStr=Bus: PRESCAN_RPY_DATA  NonVirtualBus=on
  Bus Creator3 : BusCreator  Inputs=3  OutDataTypeStr=Bus: PRESCAN_XYZ_DATA  NonVirtualBus=on
  Data Type Conversion : DataTypeConversion  OutDataTypeStr=int32  RndMeth=Nearest
  Degrees to Radians : simulink_extras/Transformations/Degrees to Radians
  Demux : Demux  Outputs=3
  Demux1 : Demux  Outputs=3
  Demux2 : Demux  Outputs=3
  Lights : Outport
  wires:
  TextureResourceID [-]/1 -> Data Type Conversion/1  "TextureResourceID"
  MSCD [Cd]/1 -> Bus Creator/1  "Intensity"
  Bus Creator/1 -> Lights/1
  Demux/1 -> Bus Creator1/1  "R"
  Demux/2 -> Bus Creator1/2  "G"
  Demux/3 -> Bus Creator1/3  "B"
  Color [-]/1 -> Demux/1  "Color"
  Bus Creator1/1 -> Bus Creator/4  "Color"
  Demux1/1 -> Bus Creator2/1  "Roll"
  Demux1/2 -> Bus Creator2/2  "Pitch"
  Demux1/3 -> Bus Creator2/3  "Yaw"
  Orientation (RPY) [deg]/1 -> Degrees to Radians/1  "Orientation"
  Bus Creator2/1 -> Bus Creator/3  "Orientation"
  Demux2/1 -> Bus Creator3/1  "X"
  Demux2/2 -> Bus Creator3/2  "Y"
  Demux2/3 -> Bus Creator3/3  "Z"
  Position (xyz) [m]/1 -> Demux2/1  "Position"
  Bus Creator3/1 -> Bus Creator/2  "Position"
  Data Type Conversion/1 -> Bus Creator/5  "TextureResourceID"
  Degrees to Radians/1 -> Demux1/1

== system TSR_Scenario_002_cs/Nissan_Cabstar_1/Indicator_side_right_Mux ==
  MSCD [Cd] : Inport
  Position (xyz) [m] : Inport  Port=2
  Orientation (RPY) [deg] : Inport  Port=3
  Color [-] : Inport  Port=4
  TextureResourceID [-] : Inport  Port=5
  Bus Creator : BusCreator  Inputs='Intensity','Position','Orientation','Color','TextureResourceID'  OutDataTypeStr=Bus: PRESCAN_VISULIGHTACTUATOR_DATA  NonVirtualBus=on
  Bus Creator1 : BusCreator  Inputs=3  OutDataTypeStr=Bus: PRESCAN_RGB_DATA  NonVirtualBus=on
  Bus Creator2 : BusCreator  Inputs=3  OutDataTypeStr=Bus: PRESCAN_RPY_DATA  NonVirtualBus=on
  Bus Creator3 : BusCreator  Inputs=3  OutDataTypeStr=Bus: PRESCAN_XYZ_DATA  NonVirtualBus=on
  Data Type Conversion : DataTypeConversion  OutDataTypeStr=int32  RndMeth=Nearest
  Degrees to Radians : simulink_extras/Transformations/Degrees to Radians
  Demux : Demux  Outputs=3
  Demux1 : Demux  Outputs=3
  Demux2 : Demux  Outputs=3
  Lights : Outport
  wires:
  TextureResourceID [-]/1 -> Data Type Conversion/1  "TextureResourceID"
  MSCD [Cd]/1 -> Bus Creator/1  "Intensity"
  Bus Creator/1 -> Lights/1
  Demux/1 -> Bus Creator1/1  "R"
  Demux/2 -> Bus Creator1/2  "G"
  Demux/3 -> Bus Creator1/3  "B"
  Color [-]/1 -> Demux/1  "Color"
  Bus Creator1/1 -> Bus Creator/4  "Color"
  Demux1/1 -> Bus Creator2/1  "Roll"
  Demux1/2 -> Bus Creator2/2  "Pitch"
  Demux1/3 -> Bus Creator2/3  "Yaw"
  Orientation (RPY) [deg]/1 -> Degrees to Radians/1  "Orientation"
  Bus Creator2/1 -> Bus Creator/3  "Orientation"
  Demux2/1 -> Bus Creator3/1  "X"
  Demux2/2 -> Bus Creator3/2  "Y"
  Demux2/3 -> Bus Creator3/3  "Z"
  Position (xyz) [m]/1 -> Demux2/1  "Position"
  Bus Creator3/1 -> Bus Creator/2  "Position"
  Data Type Conversion/1 -> Bus Creator/5  "TextureResourceID"
  Degrees to Radians/1 -> Demux1/1

== system TSR_Scenario_002_cs/Nissan_Cabstar_1/JointGroup_WheelDisplacement_V2R ==
  Velocity [m/s] : Inport  SampleTime=TimeStep
  Discrete-Time Integrator : DiscreteIntegrator  SampleTime=TimeStep
  omega=V/Rwheel : Gain  Gain=1/TireRadius
  Rotation [rad] : Outport
  wires:
  Discrete-Time Integrator/1 -> Rotation [rad]/1  "roty"
  omega=V/Rwheel/1 -> Discrete-Time Integrator/1  "rotational speed [rad/s]"
  Velocity [m/s]/1 -> omega=V/Rwheel/1

== system TSR_Scenario_002_cs/Nissan_Cabstar_1/SELF_Demux ==
  SELF : Inport  OutDataTypeStr=Bus: PRESCAN_SELFSENSORDATA
  Bus Selector : BusSelector  OutputSignals=PositionX,PositionY,PositionZ,OrientationRoll,OrientationPitch,OrientationYaw,Velocity,Yaw_rate,Lat,Long,Alt
  Demux2 : Demux  Outputs=3
  Gain : Gain  Gain=180/pi
  Gain1 : Gain  Gain=180/pi
  Vector Concatenate1 : Concatenate  NumInputs=3
  compas converter : Subsystem
  x [m] : Outport
  y [m] : Outport  Port=2
  z [m] : Outport  Port=3
  rotx [deg] : Outport  Port=4
  roty [deg] : Outport  Port=5
  rotz [deg] : Outport  Port=6
  GPS lat [deg] : Outport  Port=7
  GPS long [deg] : Outport  Port=8
  GPS alt [m] : Outport  Port=9
  velocity [m/s] : Outport  Port=10
  heading [deg] : Outport  Port=11
  yaw rate [deg/s] : Outport  Port=12
  wires:
  Bus Selector/11 -> GPS alt [m]/1  "<Alt>"
  Bus Selector/10 -> GPS long [deg]/1  "<Long>"
  Bus Selector/9 -> GPS lat [deg]/1  "<Lat>"
  Bus Selector/8 -> Gain1/1  "<Yaw_rate>"
  Bus Selector/7 -> velocity [m/s]/1  "<Velocity>"
  Bus Selector/6 -> compas converter/1(rotz [rad]), Vector Concatenate1/3  "<OrientationYaw>"
  Bus Selector/5 -> Vector Concatenate1/2  "<OrientationPitch>"
  Bus Selector/4 -> Vector Concatenate1/1  "<OrientationRoll>"
  Vector Concatenate1/1 -> Gain/1
  Bus Selector/3 -> z [m]/1  "<PositionZ>"
  Bus Selector/2 -> y [m]/1  "<PositionY>"
  Bus Selector/1 -> x [m]/1  "<PositionX>"
  SELF/1 -> Bus Selector/1
  Gain/1 -> Demux2/1
  Demux2/1 -> rotx [deg]/1
  Demux2/2 -> roty [deg]/1
  Demux2/3 -> rotz [deg]/1
  compas converter/1(heading [deg]) -> heading [deg]/1
  Gain1/1 -> yaw rate [deg/s]/1

== system TSR_Scenario_002_cs/Nissan_Cabstar_1/SteeringColumn_pivot_Mux ==
  X [m] : Inport
  Y [m] : Inport  Port=2
  Z [m] : Inport  Port=3
  Roll [rad] : Inport  Port=4
  Pitch [rad] : Inport  Port=5
  Yaw [rad] : Inport  Port=6
  Bus Creator : BusCreator  Inputs=3  OutDataTypeStr=Bus: PRESCAN_XYZ_DATA
  Bus Creator1 : BusCreator  Inputs=3  OutDataTypeStr=Bus: PRESCAN_RPY_DATA
  Bus Creator2 : BusCreator  Inputs=2  OutDataTypeStr=Bus: PRESCAN_POSE_DATA
  Joint : Outport
  wires:
  Yaw [rad]/1 -> Bus Creator1/3  "Yaw"
  Bus Creator1/1 -> Bus Creator2/2  "ORIENTATION"
  Bus Creator/1 -> Bus Creator2/1  "POSITION"
  X [m]/1 -> Bus Creator/1  "X"
  Y [m]/1 -> Bus Creator/2  "Y"
  Z [m]/1 -> Bus Creator/3  "Z"
  Bus Creator2/1 -> Joint/1
  Roll [rad]/1 -> Bus Creator1/1  "Roll"
  Pitch [rad]/1 -> Bus Creator1/2  "Pitch"

== system TSR_Scenario_002_cs/Nissan_Cabstar_1/SteeringWheel_pivot_Mux ==
  X [m] : Inport
  Y [m] : Inport  Port=2
  Z [m] : Inport  Port=3
  Roll [rad] : Inport  Port=4
  Pitch [rad] : Inport  Port=5
  Yaw [rad] : Inport  Port=6
  Bus Creator : BusCreator  Inputs=3  OutDataTypeStr=Bus: PRESCAN_XYZ_DATA
  Bus Creator1 : BusCreator  Inputs=3  OutDataTypeStr=Bus: PRESCAN_RPY_DATA
  Bus Creator2 : BusCreator  Inputs=2  OutDataTypeStr=Bus: PRESCAN_POSE_DATA
  Joint : Outport
  wires:
  Yaw [rad]/1 -> Bus Creator1/3  "Yaw"
  Bus Creator1/1 -> Bus Creator2/2  "ORIENTATION"
  Bus Creator/1 -> Bus Creator2/1  "POSITION"
  X [m]/1 -> Bus Creator/1  "X"
  Y [m]/1 -> Bus Creator/2  "Y"
  Z [m]/1 -> Bus Creator/3  "Z"
  Bus Creator2/1 -> Joint/1
  Roll [rad]/1 -> Bus Creator1/1  "Roll"
  Pitch [rad]/1 -> Bus Creator1/2  "Pitch"

== system TSR_Scenario_002_cs/Nissan_Cabstar_1/WheelDisplacement_Mux ==
  Steering Angle Front [rad] : Inport  Tag=inport/JointGroup  SampleTime=1/100  BusOutputAsStruct=on
  Steering Angle Rear [rad] : Inport  Tag=inport/JointGroup  Port=2  SampleTime=1/100  BusOutputAsStruct=on
  Rotation [rad] : Inport  Tag=inport/JointGroup  Port=3  SampleTime=1/100  BusOutputAsStruct=on
  zDisp FL [m] : Inport  Tag=inport/JointGroup  Port=4  SampleTime=1/100  BusOutputAsStruct=on
  zDisp FR [m] : Inport  Tag=inport/JointGroup  Port=5  SampleTime=1/100  BusOutputAsStruct=on
  zDisp RL [m] : Inport  Tag=inport/JointGroup  Port=6  SampleTime=1/100  BusOutputAsStruct=on
  zDisp RR [m] : Inport  Tag=inport/JointGroup  Port=7  SampleTime=1/100  BusOutputAsStruct=on
  Ground_{1..12} (12 alike) : Ground
  WheelL0_Mux : Subsystem  Tag=mux/Joint  mask(PreScan Mux Block){DisplayName=WheelL0}
      mask prompts: DisplayName "Display Name"
      mask help:
      | This block simulates a generic joint used for generic models. This joint can be enabled/disabled from the GUI.
      |
      | For more information, please click Help.
      settings: DeleteFcn=PreScanBlockDeleteFcn;
      mask Help: eval('openHelp(254)')
  WheelL1_Mux : Subsystem  Tag=mux/Joint  mask(PreScan Mux Block){DisplayName=WheelL1}
      mask prompts: DisplayName "Display Name"
      mask help:
      | This block simulates a generic joint used for generic models. This joint can be enabled/disabled from the GUI.
      |
      | For more information, please click Help.
      settings: DeleteFcn=PreScanBlockDeleteFcn;
      mask Help: eval('openHelp(254)')
  WheelR0_Mux : Subsystem  Tag=mux/Joint  mask(PreScan Mux Block){DisplayName=WheelR0}
      mask prompts: DisplayName "Display Name"
      mask help:
      | This block simulates a generic joint used for generic models. This joint can be enabled/disabled from the GUI.
      |
      | For more information, please click Help.
      settings: DeleteFcn=PreScanBlockDeleteFcn;
      mask Help: eval('openHelp(254)')
  WheelR1_Mux : Subsystem  Tag=mux/Joint  mask(PreScan Mux Block){DisplayName=WheelR1}
      mask prompts: DisplayName "Display Name"
      mask help:
      | This block simulates a generic joint used for generic models. This joint can be enabled/disabled from the GUI.
      |
      | For more information, please click Help.
      settings: DeleteFcn=PreScanBlockDeleteFcn;
      mask Help: eval('openHelp(254)')
  WheelL0_Nissan_Cabstar_1 : Outport  Tag=outport/JointActuator  OutDataTypeStr=Bus: PRESCAN_POSE_DATA  SampleTime=1/100
  WheelL1_Nissan_Cabstar_1 : Outport  Tag=outport/JointActuator  Port=2  OutDataTypeStr=Bus: PRESCAN_POSE_DATA  SampleTime=1/100
  WheelR0_Nissan_Cabstar_1 : Outport  Tag=outport/JointActuator  Port=3  OutDataTypeStr=Bus: PRESCAN_POSE_DATA  SampleTime=1/100
  WheelR1_Nissan_Cabstar_1 : Outport  Tag=outport/JointActuator  Port=4  OutDataTypeStr=Bus: PRESCAN_POSE_DATA  SampleTime=1/100
  wires:
  WheelL0_Mux/1(Joint) -> WheelL0_Nissan_Cabstar_1/1
  WheelL1_Mux/1(Joint) -> WheelL1_Nissan_Cabstar_1/1
  WheelR0_Mux/1(Joint) -> WheelR0_Nissan_Cabstar_1/1
  WheelR1_Mux/1(Joint) -> WheelR1_Nissan_Cabstar_1/1
  Steering Angle Front [rad]/1 -> WheelR0_Mux/6(Yaw [rad]), WheelL0_Mux/6(Yaw [rad])
  Steering Angle Rear [rad]/1 -> WheelR1_Mux/6(Yaw [rad]), WheelL1_Mux/6(Yaw [rad])
  Rotation [rad]/1 -> WheelR0_Mux/5(Pitch [rad]), WheelL0_Mux/5(Pitch [rad]), WheelR1_Mux/5(Pitch [rad]), WheelL1_Mux/5(Pitch [rad])
  zDisp FL [m]/1 -> WheelL0_Mux/3(Z [m])
  zDisp FR [m]/1 -> WheelR0_Mux/3(Z [m])
  zDisp RL [m]/1 -> WheelL1_Mux/3(Z [m])
  zDisp RR [m]/1 -> WheelR1_Mux/3(Z [m])
  Ground_1/1 -> WheelL0_Mux/1(X [m])
  Ground_2/1 -> WheelL0_Mux/2(Y [m])
  Ground_3/1 -> WheelL0_Mux/4(Roll [rad])
  Ground_4/1 -> WheelL1_Mux/1(X [m])
  Ground_5/1 -> WheelL1_Mux/2(Y [m])
  Ground_6/1 -> WheelL1_Mux/4(Roll [rad])
  Ground_7/1 -> WheelR0_Mux/1(X [m])
  Ground_8/1 -> WheelR0_Mux/2(Y [m])
  Ground_9/1 -> WheelR0_Mux/4(Roll [rad])
  Ground_10/1 -> WheelR1_Mux/1(X [m])
  Ground_11/1 -> WheelR1_Mux/2(Y [m])
  Ground_12/1 -> WheelR1_Mux/4(Roll [rad])

== system TSR_Scenario_002_cs/Nissan_Cabstar_2/SELF_Demux ==
  SELF : Inport  OutDataTypeStr=Bus: PRESCAN_SELFSENSORDATA
  Bus Selector : BusSelector  OutputSignals=PositionX,PositionY,PositionZ,OrientationRoll,OrientationPitch,OrientationYaw,Velocity,Yaw_rate,Lat,Long,Alt
  Demux2 : Demux  Outputs=3
  Gain : Gain  Gain=180/pi
  Gain1 : Gain  Gain=180/pi
  Vector Concatenate1 : Concatenate  NumInputs=3
  compas converter : Subsystem
  x [m] : Outport
  y [m] : Outport  Port=2
  z [m] : Outport  Port=3
  rotx [deg] : Outport  Port=4
  roty [deg] : Outport  Port=5
  rotz [deg] : Outport  Port=6
  GPS lat [deg] : Outport  Port=7
  GPS long [deg] : Outport  Port=8
  GPS alt [m] : Outport  Port=9
  velocity [m/s] : Outport  Port=10
  heading [deg] : Outport  Port=11
  yaw rate [deg/s] : Outport  Port=12
  wires:
  Bus Selector/11 -> GPS alt [m]/1  "<Alt>"
  Bus Selector/10 -> GPS long [deg]/1  "<Long>"
  Bus Selector/9 -> GPS lat [deg]/1  "<Lat>"
  Bus Selector/8 -> Gain1/1  "<Yaw_rate>"
  Bus Selector/7 -> velocity [m/s]/1  "<Velocity>"
  Bus Selector/6 -> compas converter/1(rotz [rad]), Vector Concatenate1/3  "<OrientationYaw>"
  Bus Selector/5 -> Vector Concatenate1/2  "<OrientationPitch>"
  Bus Selector/4 -> Vector Concatenate1/1  "<OrientationRoll>"
  Vector Concatenate1/1 -> Gain/1
  Bus Selector/3 -> z [m]/1  "<PositionZ>"
  Bus Selector/2 -> y [m]/1  "<PositionY>"
  Bus Selector/1 -> x [m]/1  "<PositionX>"
  SELF/1 -> Bus Selector/1
  Gain/1 -> Demux2/1
  Demux2/1 -> rotx [deg]/1
  Demux2/2 -> roty [deg]/1
  Demux2/3 -> rotz [deg]/1
  compas converter/1(heading [deg]) -> heading [deg]/1
  Gain1/1 -> yaw rate [deg/s]/1

== system TSR_Scenario_002_cs/Nissan_Cabstar_3/Dynamics_Empty ==
  note: For state mode 'Dynamic' positions
      | are not taken into account, as they
      | are computed by integrating velocity.
      | Click annotation for Help.
  Ground_{1..9} (9 alike) : Ground
  MuxState : Subsystem  Tag=mux/State  mask(Empty Dynamics State Block){positioningmode=on, TimeStep=1/100}
      mask prompts: positioningmode "Positioning Mode"; TimeStep "Auto Assigned: Time Step [s]"
      mask help:
      | Build the state of an actor based on user input.
      | The user can either use positioning mode or dynamics mode.
      | - When using positioning mode the position and orientation of the actor are set directly based on the input. Expected input is relative to the initial position and orientation of the actor. It's also possible to specify the velocity of the actor, though this input isn't used, only passed on.
      | - When using dynamics mode the position input is ignored. Expected input is velocity and orientation. The velocity is relative the current orientation of the actor, while orientation is relative to its initial orientation. The position of the actor is calculated based on the velocity and orientation given.
      settings: DeleteFcn=PreScanBlockDeleteFcn;
  STATE_Nissan_Cabstar_3 : Subsystem  Tag=mux/StatePort  Priority=0  LoadFcn=load PrescanStateActuatorData  mask(PreScan Sink Block: State){x0=TSR_Scenario_002_cs_70c7e369ce6550e0, y0=TSR_Scenario_002_cs_538caacf3455966d, z0=TSR_Scenario_002_cs_4dd419d6d2b56fc2, Roll0=TSR_Scenario_002_cs_3460ff54d38ab2e2, Pitch0=TSR_Scenario_002_cs_2ac3337370d0049d, Yaw0=TSR_Scenario_002_cs_1e339fa5d680f213, TimeStep=1/100}
      mask prompts: x0 "Ini x-position VEHICLE wrt GLOBAL axis system [m]"; y0 "Ini y-position VEHICLE wrt GLOBAL axis system [m]"; z0 "Ini z-position VEHICLE wrt GLOBAL axis system [m]"; Roll0 "Ini roll-angle BODY wrt VEHICLE axis system [deg]"; Pitch0 "Ini pitch-angle BODY wrt VEHICLE axis system [deg]"; Yaw0 "Ini yaw-angle VEHICLE wrt GLOBAL axis system [deg]"; TimeStep "Auto-Assigned: Upload Period [s]"
      mask help:
      | The Actor State contains a vector signal of size (9x1), containing the following signals:
      |
      | -  Position                  (x,y,z)                                     [m]
      | -  Velocity                  (vx,vy,vz)                               [m/s]
      | -  Angles                    (Roll, Pitch, Yaw)                   [rad]
      |
      | The Actor state is defined in the global axis system.
      | The state is superponed on the Initial position defined in the GUI.
      |
      | For more information, please click Help.
      settings: DeleteFcn=PreScanBlockDeleteFcn;
      mask Help: eval('openHelp(222)')
      mask Display: image(imread('State.png'))
  State : Outport  Tag=outport/StateOutport  SampleTime=1/100
  wires:
  MuxState/1(state) -> STATE_Nissan_Cabstar_3/1(State)
  STATE_Nissan_Cabstar_3/1(StateBus) -> State/1
  Ground_1/1 -> MuxState/1(x [m])
  Ground_2/1 -> MuxState/2(y [m])
  Ground_3/1 -> MuxState/3(z [m])
  Ground_4/1 -> MuxState/4(dx [m/s])
  Ground_5/1 -> MuxState/5(dy [m/s])
  Ground_6/1 -> MuxState/6(dz [m/s])
  Ground_7/1 -> MuxState/7(R [rad])
  Ground_8/1 -> MuxState/8(P [rad])
  Ground_9/1 -> MuxState/9(Y [rad])

== system TSR_Scenario_002_cs/Nissan_Cabstar_3/SELF_Demux ==
  SELF : Inport  OutDataTypeStr=Bus: PRESCAN_SELFSENSORDATA
  Bus Selector : BusSelector  OutputSignals=PositionX,PositionY,PositionZ,OrientationRoll,OrientationPitch,OrientationYaw,Velocity,Yaw_rate,Lat,Long,Alt
  Demux2 : Demux  Outputs=3
  Gain : Gain  Gain=180/pi
  Gain1 : Gain  Gain=180/pi
  Vector Concatenate1 : Concatenate  NumInputs=3
  compas converter : Subsystem
  x [m] : Outport
  y [m] : Outport  Port=2
  z [m] : Outport  Port=3
  rotx [deg] : Outport  Port=4
  roty [deg] : Outport  Port=5
  rotz [deg] : Outport  Port=6
  GPS lat [deg] : Outport  Port=7
  GPS long [deg] : Outport  Port=8
  GPS alt [m] : Outport  Port=9
  velocity [m/s] : Outport  Port=10
  heading [deg] : Outport  Port=11
  yaw rate [deg/s] : Outport  Port=12
  wires:
  Bus Selector/11 -> GPS alt [m]/1  "<Alt>"
  Bus Selector/10 -> GPS long [deg]/1  "<Long>"
  Bus Selector/9 -> GPS lat [deg]/1  "<Lat>"
  Bus Selector/8 -> Gain1/1  "<Yaw_rate>"
  Bus Selector/7 -> velocity [m/s]/1  "<Velocity>"
  Bus Selector/6 -> compas converter/1(rotz [rad]), Vector Concatenate1/3  "<OrientationYaw>"
  Bus Selector/5 -> Vector Concatenate1/2  "<OrientationPitch>"
  Bus Selector/4 -> Vector Concatenate1/1  "<OrientationRoll>"
  Vector Concatenate1/1 -> Gain/1
  Bus Selector/3 -> z [m]/1  "<PositionZ>"
  Bus Selector/2 -> y [m]/1  "<PositionY>"
  Bus Selector/1 -> x [m]/1  "<PositionX>"
  SELF/1 -> Bus Selector/1
  Gain/1 -> Demux2/1
  Demux2/1 -> rotx [deg]/1
  Demux2/2 -> roty [deg]/1
  Demux2/3 -> rotz [deg]/1
  compas converter/1(heading [deg]) -> heading [deg]/1
  Gain1/1 -> yaw rate [deg/s]/1
